simulink model "OpenLoopPosition"  (R2019a)
settings: Solver=VariableStepAuto  StartTime=0.0  StopTime=10.0  RelTol=1e-3
values from neighbouring files (symbols this model uses):
  den2 = [1 47.56 1309]    [BallandBeamModeling.m]
  num2 = [5.94e04]    [BallandBeamModeling.m]
undefined symbols (not defined in the file or in its folder): Kdin, Kdout, Kiout, Kpin, Kpout
settings Model: Creator=xde12  LastModifiedBy=xde12

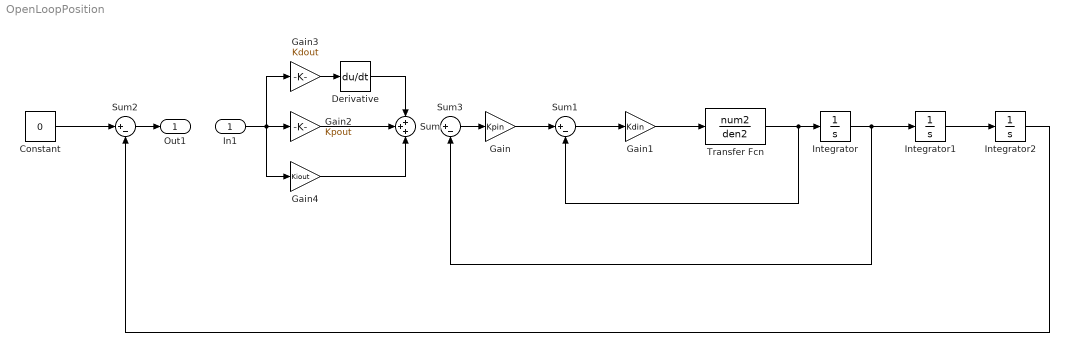
== system OpenLoopPosition ==
  In1 : Inport
  Constant : Constant  Value=0
  Derivative : Derivative
  Gain : Gain  Gain=Kpin
  Gain1 : Gain  Gain=Kdin
  Gain2 : Gain  Gain=Kpout
  Gain3 : Gain  Gain=Kdout
  Gain4 : Gain  Gain=Kiout
  Integrator : Integrator
  Integrator1 : Integrator
  Integrator2 : Integrator
  Sum : Sum  Inputs=+++
  Sum1 : Sum  Inputs=|+-
  Sum2 : Sum  Inputs=|+-
  Sum3 : Sum  Inputs=|+-
  Transfer Fcn : TransferFcn  Numerator=num2  Denominator=den2
  Out1 : Outport
  wires:
  Gain/1 -> Sum1/1
  Sum1/1 -> Gain1/1
  Gain1/1 -> Transfer Fcn/1
  Transfer Fcn/1 -> Sum1/2, Integrator/1
  Gain2/1 -> Sum/2
  Gain3/1 -> Derivative/1
  Derivative/1 -> Sum/1
  Integrator1/1 -> Integrator2/1
  Integrator2/1 -> Sum2/2
  Constant/1 -> Sum2/1
  In1/1 -> Gain4/1, Gain3/1, Gain2/1
  Sum2/1 -> Out1/1
  Sum3/1 -> Gain/1
  Integrator/1 -> Integrator1/1, Sum3/2
  Gain4/1 -> Sum/3
